simulink model "deney4_3"  (R2025b)
settings: Solver=VariableStepAuto  StartTime=0.0  StopTime=10.0  RelTol=1e-3
settings Model: Creator=Seyma  LastModifiedBy=Seyma

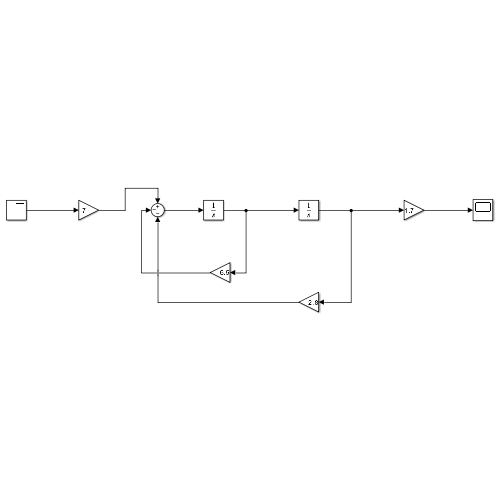
[thumbnail: Simulink's stored preview of the top-level diagram]
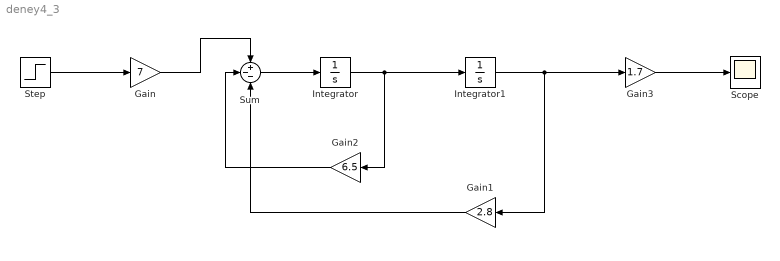
== system deney4_3 ==
  Gain : Gain  Gain=7
  Gain1 : Gain  Gain=2.8
  Gain2 : Gain  Gain=6.5
  Gain3 : Gain  Gain=1.7
  Integrator : Integrator
  Integrator1 : Integrator
  Scope : Scope
      settings: ActiveDisplayYMinimum=-0.52568521010278713  ActiveDisplayYMaximum=4.7311668909250848
  Step : Step  Time=0  SampleTime=0
  Sum : Sum  Inputs=+--
  wires:
  Step/1 -> Gain/1
  Sum/1 -> Integrator/1
  Gain/1 -> Sum/1
  Integrator/1 -> Integrator1/1, Gain2/1
  Gain2/1 -> Sum/2
  Integrator1/1 -> Gain3/1, Gain1/1
  Gain1/1 -> Sum/3
  Gain3/1 -> Scope/1
